simulink model "CMU_BORG_AplysiaModularNeuromechanics"  (R2024a)
settings: Solver=ode23  StartTime=0.0  StopTime=tend  FixedStep=0.001  MaxStep=0.1  RelTol=0.00001  AbsTol=0.0001
values from neighbouring files (symbols this model uses):
  B20_0 = 0    [ParameterRecalculation.m]    (also in ReferenceGeometry_and_Initialization.m)
  B31B32_0 = 0    [GetSteadyState.m]    (also in ParameterRecalculation.m = 1; ReferenceGeometry_and_Initialization.m = 1; VaryingSeaweedStrength.m = 1)
  B38_0 = 0    [ParameterRecalculation.m]    (also in ReferenceGeometry_and_Initialization.m)
  B40B30_0 = 0    [ParameterRecalculation.m]    (also in ReferenceGeometry_and_Initialization.m)
  B40B30_offTime_0 = 0    [ParameterRecalculation.m]    (also in ReferenceGeometry_and_Initialization.m)
  B43B45_0 = 0    [ParameterRecalculation.m]    (also in ReferenceGeometry_and_Initialization.m)
  B4B5_0 = 0    [ParameterRecalculation.m]    (also in ReferenceGeometry_and_Initialization.m)
  B64_0 = 1    [GetSteadyState.m]    (also in ParameterRecalculation.m = 0; ReferenceGeometry_and_Initialization.m = 0; VaryingSeaweedStrength.m = 0)
  B6B9B3_0 = 1    [GetSteadyState.m]    (also in ParameterRecalculation.m = 0; ReferenceGeometry_and_Initialization.m = 0; VaryingSeaweedStrength.m = 0)
  B7_0 = 0    [ParameterRecalculation.m]    (also in ReferenceGeometry_and_Initialization.m)
  B8_0 = 0    [ParameterRecalculation.m]    (also in ReferenceGeometry_and_Initialization.m)
  C1_0 = 0    [ParameterRecalculation.m]    (also in ReferenceGeometry_and_Initialization.m)
  C2_0 = 0    [ParameterRecalculation.m]    (also in ReferenceGeometry_and_Initialization.m)
  C6_0 = 0    [ParameterRecalculation.m]    (also in ReferenceGeometry_and_Initialization.m)
  C_theta = C_xg/(2*pi)    [ParameterRecalculation.m]    (also in ReferenceGeometry_and_Initialization.m = 0.000813600069086)
  C_xd = C_xg    [ParameterRecalculation.m]    (also in ReferenceGeometry_and_Initialization.m = 0.005112)
  C_xg = (1/inv_C(kk))*time_scaler*force_scaler    [DampingParameterConvergence.m]    (also in ReferenceGeometry_and_Initialization.m = 0.005112)
  C_xv = C_xd    [ParameterRecalculation.m]    (also in ReferenceGeometry_and_Initialization.m = 0.005112)
  C_yg = C_xg    [ParameterRecalculation.m]    (also in ReferenceGeometry_and_Initialization.m = 0.005112)
  CBI2_0 = 0    [ParameterRecalculation.m]    (also in ReferenceGeometry_and_Initialization.m)
  CBI3_0 = 0    [GetSteadyState.m]    (also in ParameterRecalculation.m = 1; ReferenceGeometry_and_Initialization.m = 1; VaryingSeaweedStrength.m = 1)
  CBI3_refractory_0 = 0    [ParameterRecalculation.m]    (also in ReferenceGeometry_and_Initialization.m)
  CBI3_stimOFF_0 = 0    [ParameterRecalculation.m]    (also in ReferenceGeometry_and_Initialization.m)
  CBI3_stimON_0 = 0    [ParameterRecalculation.m]    (also in ReferenceGeometry_and_Initialization.m)
  CBI4_0 = 0    [ParameterRecalculation.m]    (also in ReferenceGeometry_and_Initialization.m)
  E1_params = [AE10,TE10,tau_E1,L0_E1,Lmax_E1]    [ParameterRecalculation.m]    (also in ReferenceGeometry_and_Initialization.m)
  E2_params = [AE20,TE20,tau_E2,L0_E2,Lmax_E2]    [ParameterRecalculation.m]    (also in ReferenceGeometry_and_Initialization.m)
  E6_params = [AE60,TE60,tau_E6,L0_E6,Lmax_E6]    [ParameterRecalculation.m]    (also in ReferenceGeometry_and_Initialization.m)
  FE1_max = force_scaler*0.2    [ParameterRecalculation.m]    (also in ReferenceGeometry_and_Initialization.m = 0.048)
  FE2_max = FE1_max    [ParameterRecalculation.m]    (also in ReferenceGeometry_and_Initialization.m = 0.048)
  FE6_max = FE1_max    [ParameterRecalculation.m]    (also in ReferenceGeometry_and_Initialization.m = 0.048)
  FHinge_max = force_scaler*0.292    [ParameterRecalculation.m]    (also in ReferenceGeometry_and_Initialization.m = 0.07008)
  FI1d_max = force_scaler*3.2    [ParameterRecalculation.m]    (also in ReferenceGeometry_and_Initialization.m = 0.768)
  FI1v_max = FI1d_max    [ParameterRecalculation.m]    (also in ReferenceGeometry_and_Initialization.m = 0.768)
  FI2_max = force_scaler*1    [ParameterRecalculation.m]    (also in ReferenceGeometry_and_Initialization.m = 0.24)
  FI3_ant_max = force_scaler*0.1    [ParameterRecalculation.m]    (also in ReferenceGeometry_and_Initialization.m = 0.024)
  FI3_max = force_scaler*3    [ParameterRecalculation.m]    (also in ReferenceGeometry_and_Initialization.m = 0.72)
  FI4_max = force_scaler*0.9    [ParameterRecalculation.m]    (also in ReferenceGeometry_and_Initialization.m = 0.216)
  fixation_type = 0    [GetSteadyState.m]    (also in ModelController.m; VaryingSeaweedStrength.m)
  grasperR = 1    [ReferenceGeometry_and_Initialization.m]
  H_lumen = mean([L_jaw,L_LG]) / R_ref    [ReferenceGeometry_and_Initialization.m]
  Hinge_params = [A_hinge0,T_hinge0,tau_hinge,L0_hinge,Lmax_hinge]    [ParameterRecalculation.m]    (also in ReferenceGeometry_and_Initialization.m)
  I1d_params = [AI1d0,TI1d0,tau_I1d,L0_I1d,Lmax_I1d]    [ParameterRecalculation.m]    (also in ReferenceGeometry_and_Initialization.m)
  I1v_params = [AI1v0,TI1v0,tau_I1v,L0_I1v,Lmax_I1v]    [ParameterRecalculation.m]    (also in ReferenceGeometry_and_Initialization.m)
  I2_params = [AI20,TI20,tau_I2_ingestive,tau_I2_egestive,L0_I2,Lmax_I2]    [ParameterRecalculation.m]    (also in ReferenceGeometry_and_Initialization.m)
  I3_params = [AI30,TI30,tau_I3]    [ParameterRecalculation.m]    (also in ReferenceGeometry_and_Initialization.m)
  I3ant_params = [AI3_ant0,TI3_ant0,tau_I3ant]    [ParameterRecalculation.m]    (also in ReferenceGeometry_and_Initialization.m)
  I4_params = [AI40,TI40,tau_I4]    [ParameterRecalculation.m]    (also in ReferenceGeometry_and_Initialization.m)
  K_const = force_scaler*0.5    [ParameterRecalculation.m]    (also in ReferenceGeometry_and_Initialization.m = 0.12)
  K_Eso = force_scaler*0.01    [ParameterRecalculation.m]    (also in ReferenceGeometry_and_Initialization.m = 0.0024)
  K_H = force_scaler*2    [ParameterRecalculation.m]    (also in ReferenceGeometry_and_Initialization.m = 0.48)
  L0_eso = abs(xd0)    [ReferenceGeometry_and_Initialization.m]
  L0_H = 0    [ReferenceGeometry_and_Initialization.m]
  L0_I1d = L1d0    [ParameterRecalculation.m]    (also in ReferenceGeometry_and_Initialization.m)
  L0_I1v = L1v0    [ParameterRecalculation.m]    (also in ReferenceGeometry_and_Initialization.m)
  L_head = 0.82*tracing_scale_factor    [ReferenceGeometry_and_Initialization.m]
  MCC_0 = 1    [DampingParameterConvergence.m]    (also in ModelController.m; ParameterRecalculation.m = 0; ReferenceGeometry_and_Initialization.m = 0)
  params = param_vec    [ParameterRecalculation.m]    (also in ReferenceGeometry_and_Initialization.m)
  seaweed_strength = 1e6    (= 1000000)    [ModelController.m]    (also in VaryingSeaweedStrength.m = seaweed_strength_vec(ind))
  sens_chemical_lips = 0    [GetSteadyState.m]    (also in ModelController.m = 1; VaryingSeaweedStrength.m = 1)
  sens_mechanical_grasper = 1    [GetSteadyState.m]    (also in ModelController.m = 0; VaryingSeaweedStrength.m)
  sens_mechanical_lips = 1    [GetSteadyState.m]    (also in ModelController.m; VaryingSeaweedStrength.m)
  t_switch_chem_lips = 1e6    (= 1000000)    [GetSteadyState.m]    (also in ModelController.m = 54; VaryingSeaweedStrength.m)
  t_switch_fixation = 1e6    (= 1000000)    [GetSteadyState.m]    (also in ModelController.m = 30; VaryingSeaweedStrength.m = 4)
  t_switch_mech_grasp = 1e6    (= 1000000)    [GetSteadyState.m]    (also in ModelController.m = 10; VaryingSeaweedStrength.m)
  t_switch_mech_lips = 1e6    (= 1000000)    [GetSteadyState.m]    (also in ModelController.m; VaryingSeaweedStrength.m)
  theta_fg = buccal_mass_data(7)    [PlotModel.m]    (also in ReferenceGeometry_and_Initialization.m = -(head_outline{4,"Angle"} - head_outline{3,"Angle"})*(pi/180)
  theta_g0 = (180-(head_outline{3,"Angle"} + rot_global +5))*(pi/180)    [ReferenceGeometry_and_Initialization.m]
  theta_H = buccal_mass_data(6)    [PlotModel.m]    (also in ReferenceGeometry_and_Initialization.m = pi + theta_H_tilde - theta_g0)
  time_scaler = 1    [DampingParameterConvergence.m]    (also in ReferenceGeometry_and_Initialization.m = 1.065)
  ukg = 0.95*usg    (= 0.95)    [ParameterRecalculation.m]    (also in ReferenceGeometry_and_Initialization.m)
  ukh = 0.75*ush    (= 0.75)    [ParameterRecalculation.m]    (also in ReferenceGeometry_and_Initialization.m)
  usg = 1    [ParameterRecalculation.m]    (also in ReferenceGeometry_and_Initialization.m)
  ush = 1    [ParameterRecalculation.m]    (also in ReferenceGeometry_and_Initialization.m)
  xd0 = L_head - L1d0    [ReferenceGeometry_and_Initialization.m]
  xg0 = L_head + L_CG * cosd(a_CG) + 0.3    [ReferenceGeometry_and_Initialization.m]
  xh0 = 0    [ReferenceGeometry_and_Initialization.m]
  xv0 = L_head - L1v0    [ReferenceGeometry_and_Initialization.m]
  yg0 = L_CG * sind(a_CG) + 0.4    [ReferenceGeometry_and_Initialization.m]
(part 1 of 4)
settings Model: SimulationMode=accelerator  Creator=MichaelBennington  LastModifiedBy=MichaelBennington
settings SolverCC: ZeroCrossControl=DisableAll  ZeroCrossAlgorithm=Adaptive
settings OptimizationCC: ReuseModelBlockBuffer=off
settings DebuggingCC: IgnoredZcDiagnostic=none
settings RTWCC: GPUComputeCapability=3.5

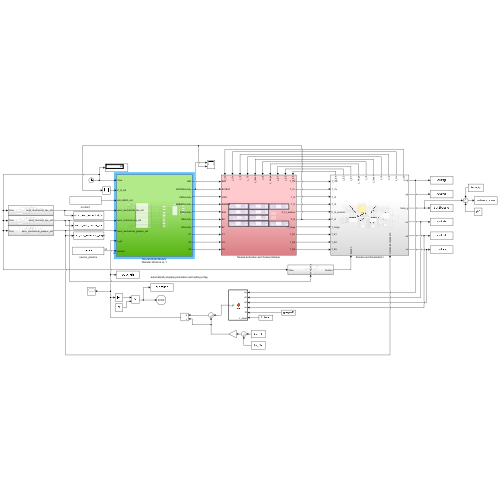
[thumbnail: Simulink's stored preview of the top-level diagram]
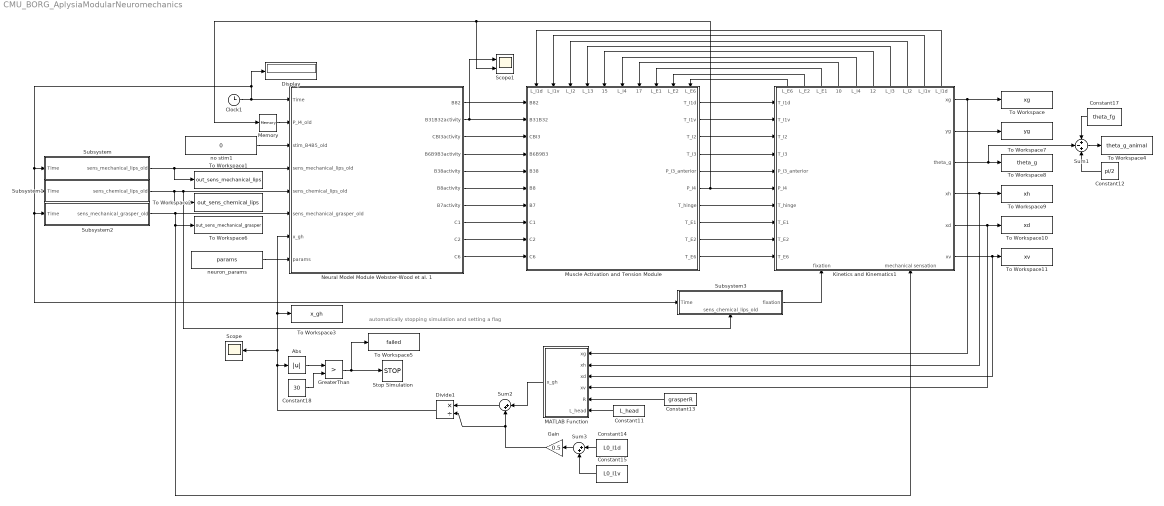
== system CMU_BORG_AplysiaModularNeuromechanics ==
  note: automatically stopping simulation and setting a flag
  Abs : Abs  SaturateOnIntegerOverflow=off
  Clock1 : Clock
  Constant11 : Constant  Value=L_head
  Constant12 : Constant  Value=pi/2
  Constant13 : Constant  Value=grasperR
  Constant14 : Constant  Value=L0_I1d
  Constant15 : Constant  Value=L0_I1v
  Constant17 : Constant  Value=theta_fg
  Constant18 : Constant  Value=30
  Display : Display
  Divide1 : Product  Inputs=*/
  Gain : Gain  Gain=0.5
  GreaterThan : RelationalOperator  Operator=>  OutDataTypeStr=boolean  RndMeth=Simplest  InputSameDT=off
  Kinetics and Kinematics1 : Subsystem
      settings: PortSchema="{\"entries\":[{\"content\":{\"sides\":[{\"content\":{\"connectorIds\":[\"In1\",\"In2\",\"In3\",\"In4\",\"In5\",\"In6\",\"In7\",\"In8\",\"In9\",\"In10\"]},\"type\":\"ConnectorPlacement.EquallySpacedRectSide\",\"uuid\":\"feb973b9-0be4-4875-8bab-e7ecafe4ce91\"},{\"content\":{\"connectorIds\":[\"Out1\",\"Out2\",\"Out3\",\"Out4\",\"Out5\",\"Out6\"],\"side\":\"RIGHT\"},\"type\":\"ConnectorPlacement.EquallySpacedRectSide\",\"uuid\":\"c5092c36-404e-4254-bef3-0d67bb5be9d9\"},{\"content\":{\"connectorIds\":[\"Out7\",\"Out8\",\"Out9\",\"Out10\",\"Out11\",\"Out12\",\"Out13\",\"Out14\",\"Out15\",\"Out16\"],\"side\":\"TOP\"},\"type\":\"ConnectorPlacement.EquallySpacedRectSide\",\"uuid\":\"bd9119a0-4095-4707-a24a-63f80d66a5e2\"},{\"content\":{\"connectorIds\":[\"In11\",\"In12\"],\"side\":\"BOTTOM\"},\"type\":\"ConnectorPlacement.EquallySpacedRectSide\",\"uuid\":\"ad89abb6-7f53-48b7-b4f1-a6034e6f6b49\"}]},\"type\":\"ConnectorPlacement.EquallySpacedConnector\",\"uuid\":\"6bece42c-f05e-4dc2-8f2f-f52897a5dfb1\"}],\"packageUris\":[\"http://schema.mathworks.com/mf0/Connector/R2020b\"],\"version\":\"1.0\"}"
  MATLAB Function : MATLAB Function  TreatAsAtomicUnit=on
  Memory : Memory
  Muscle Activation and Tension Module : Subsystem
      settings: PortSchema="{\"entries\":[{\"content\":{\"sides\":[{\"content\":{\"connectorIds\":[\"In1\",\"In2\",\"In3\",\"In4\",\"In5\",\"In6\",\"In7\",\"In8\",\"In9\",\"In10\"]},\"type\":\"ConnectorPlacement.EquallySpacedRectSide\",\"uuid\":\"3ed42070-edfc-4f7d-bbc9-5418b4631d85\"},{\"content\":{\"connectorIds\":[\"Out1\",\"Out2\",\"Out3\",\"Out4\",\"Out5\",\"Out6\",\"Out7\",\"Out8\",\"Out9\",\"Out10\"],\"side\":\"RIGHT\"},\"type\":\"ConnectorPlacement.EquallySpacedRectSide\",\"uuid\":\"9529d621-06eb-4de0-be68-068c8ead65ac\"},{\"content\":{\"connectorIds\":[\"In11\",\"In12\",\"In13\",\"In14\",\"In15\",\"In16\",\"In17\",\"In18\",\"In19\",\"In20\"],\"side\":\"TOP\"},\"type\":\"ConnectorPlacement.EquallySpacedRectSide\",\"uuid\":\"028e6ff9-8ac1-449c-b22e-a0a954505d61\"}]},\"type\":\"ConnectorPlacement.EquallySpacedConnector\",\"uuid\":\"edcba6fa-e4ae-48e3-a50b-df7cd108ff35\"}],\"packageUris\":[\"http://schema.mathworks.com/mf0/Connector/R2020b\"],\"version\":\"1.0\"}"
  Neural Model Module Webster-Wood et al. 1 : Subsystem
  Scope : Scope
  Scope1 : Scope  NumInputPorts=2
  Stop Simulation : Stop
  Subsystem : Subsystem
  Subsystem1 : Subsystem
  Subsystem2 : Subsystem
  Subsystem3 : Subsystem
      settings: PortSchema="{\"entries\":[{\"content\":{\"sides\":[{\"content\":{\"connectorIds\":[\"In1\"]},\"type\":\"ConnectorPlacement.EquallySpacedRectSide\",\"uuid\":\"4db34430-399f-4704-aacb-c58121948b76\"},{\"content\":{\"connectorIds\":[\"Out1\"],\"side\":\"RIGHT\"},\"type\":\"ConnectorPlacement.EquallySpacedRectSide\",\"uuid\":\"b1912424-5bc4-479d-9601-ca1764a05c0d\"},{\"content\":{\"connectorIds\":[],\"side\":\"TOP\"},\"type\":\"ConnectorPlacement.EquallySpacedRectSide\",\"uuid\":\"e34c704c-48ea-4069-bc3f-08ffaf2b3e65\"},{\"content\":{\"connectorIds\":[\"In2\"],\"side\":\"BOTTOM\"},\"type\":\"ConnectorPlacement.EquallySpacedRectSide\",\"uuid\":\"845d24db-429a-4efd-80d9-e92f93226b00\"}]},\"type\":\"ConnectorPlacement.EquallySpacedConnector\",\"uuid\":\"7cfd80de-20d7-4cb7-a610-d527eb736c28\"}],\"packageUris\":[\"http://schema.mathworks.com/mf0/Connector/R2020b\"],\"version\":\"1.0\"}"
  Sum1 : Sum  Inputs=+-+
  Sum2 : Sum  Inputs=|++
  Sum3 : Sum  Inputs=|++
  To Workspace : ToWorkspace  VariableName=xg  SampleTime=-1
  To Workspace1 : ToWorkspace  VariableName=out_sens_mechanical_lips  SampleTime=-1
  To Workspace10 : ToWorkspace  VariableName=xd  SampleTime=-1
  To Workspace11 : ToWorkspace  VariableName=xv  SampleTime=-1
  To Workspace2 : ToWorkspace  VariableName=out_sens_chemical_lips  SampleTime=-1
  To Workspace3 : ToWorkspace  VariableName=x_gh  SampleTime=-1
  To Workspace4 : ToWorkspace  VariableName=theta_g_animal  SampleTime=-1
  To Workspace5 : ToWorkspace  VariableName=failed  SampleTime=-1
  To Workspace6 : ToWorkspace  VariableName=out_sens_mechanical_grasper  SampleTime=-1
  To Workspace7 : ToWorkspace  VariableName=yg  SampleTime=-1
  To Workspace8 : ToWorkspace  VariableName=theta_g  SampleTime=-1
  To Workspace9 : ToWorkspace  VariableName=xh  SampleTime=-1
  neuron_params : Constant  Value=params
  no stim1 : Constant  Value=0
  wires:
  no stim1/1 -> Neural Model Module Webster-Wood et al. 1/3(stim_B4B5_old)
  Subsystem2/1(sens_mechanical_grasper_old) -> To Workspace6/1, Kinetics and Kinematics1/12(mechanical sensation), Neural Model Module Webster-Wood et al. 1/6(sens_mechanical_grasper_old)
  Subsystem3/1(fixation) -> Kinetics and Kinematics1/11(fixation)
  Kinetics and Kinematics1/7(L_E6) -> Muscle Activation and Tension Module/20(L_E6)
  Kinetics and Kinematics1/8(L_E2) -> Muscle Activation and Tension Module/19(L_E2)
  Kinetics and Kinematics1/9(L_E1) -> Muscle Activation and Tension Module/18(L_E1)
  Kinetics and Kinematics1/10(L_hinge) -> Muscle Activation and Tension Module/17(L_hinge)
  Kinetics and Kinematics1/11(L_I4) -> Muscle Activation and Tension Module/16(L_I4)
  Kinetics and Kinematics1/12(L_I3ant) -> Muscle Activation and Tension Module/15(L_I3ant)
  Kinetics and Kinematics1/13(L_I3) -> Muscle Activation and Tension Module/14(L_13)
  Kinetics and Kinematics1/14(L_I2) -> Muscle Activation and Tension Module/13(L_I2)
  Kinetics and Kinematics1/15(L_I1v) -> Muscle Activation and Tension Module/12(L_I1v)
  Kinetics and Kinematics1/16(L_I1d) -> Muscle Activation and Tension Module/11(L_I1d)
  Clock1/1 -> Subsystem1/1(Time), Subsystem3/1(Time), Subsystem2/1(Time), Subsystem/1(Time), Display/1, Neural Model Module Webster-Wood et al. 1/1(Time)
  Memory/1 -> Neural Model Module Webster-Wood et al. 1/2(P_I4_old)
  Kinetics and Kinematics1/1(xg) -> To Workspace/1, MATLAB Function/1(xg)
  Kinetics and Kinematics1/2(yg) -> To Workspace7/1
  Kinetics and Kinematics1/3(theta_g) -> Sum1/2, To Workspace8/1
  Kinetics and Kinematics1/4(xh) -> MATLAB Function/2(xh), To Workspace9/1
  Kinetics and Kinematics1/5(xd) -> MATLAB Function/4(xv), To Workspace10/1
  Kinetics and Kinematics1/6(xv) -> MATLAB Function/3(xd), To Workspace11/1
  Muscle Activation and Tension Module/1(T_I1d) -> Kinetics and Kinematics1/1(T_I1d)
  Muscle Activation and Tension Module/2(T_I1v) -> Kinetics and Kinematics1/2(T_I1v)
  Muscle Activation and Tension Module/3(T_I2) -> Kinetics and Kinematics1/3(T_I2)
  Muscle Activation and Tension Module/4(T_I3) -> Kinetics and Kinematics1/4(T_I3)
  Muscle Activation and Tension Module/5(P_I3_anterior) -> Kinetics and Kinematics1/5(P_I3_anterior)
  Muscle Activation and Tension Module/6(P_I4) -> Kinetics and Kinematics1/6(P_I4), Scope1/2, Memory/1
  Muscle Activation and Tension Module/7(T_hinge) -> Kinetics and Kinematics1/7(T_hinge)
  Muscle Activation and Tension Module/8(T_E1) -> Kinetics and Kinematics1/8(T_E1)
  Muscle Activation and Tension Module/9(T_E2) -> Kinetics and Kinematics1/9(T_E2)
  Muscle Activation and Tension Module/10(T_E6) -> Kinetics and Kinematics1/10(T_E6)
  Neural Model Module Webster-Wood et al. 1/2(B31B32activity) -> Scope1/1, Muscle Activation and Tension Module/2(B31B32)
  Neural Model Module Webster-Wood et al. 1/3(CBI3activity) -> Muscle Activation and Tension Module/3(CBI3)
  Neural Model Module Webster-Wood et al. 1/4(B6B9B3activity) -> Muscle Activation and Tension Module/4(B6B9B3)
  Neural Model Module Webster-Wood et al. 1/5(B38activity) -> Muscle Activation and Tension Module/5(B38)
  Neural Model Module Webster-Wood et al. 1/6(B8activity) -> Muscle Activation and Tension Module/6(B8)
  Neural Model Module Webster-Wood et al. 1/7(B7activity) -> Muscle Activation and Tension Module/7(B7)
  Neural Model Module Webster-Wood et al. 1/1(B82) -> Muscle Activation and Tension Module/1(B82)
  Neural Model Module Webster-Wood et al. 1/10(C6) -> Muscle Activation and Tension Module/10(C6)
  Neural Model Module Webster-Wood et al. 1/9(C2) -> Muscle Activation and Tension Module/9(C2)
  Neural Model Module Webster-Wood et al. 1/8(C1) -> Muscle Activation and Tension Module/8(C1)
  Constant11/1 -> MATLAB Function/6(L_head)
  Constant13/1 -> MATLAB Function/5(R)
  Constant14/1 -> Sum3/1
  Constant15/1 -> Sum3/2
  Sum3/1 -> Gain/1
  Sum2/1 -> Divide1/1
  Divide1/1 -> Neural Model Module Webster-Wood et al. 1/7(x_gh), To Workspace3/1, Scope/1, Abs/1
  Gain/1 -> Sum2/2, Divide1/2
  MATLAB Function/1(x_gh) -> Sum2/1
  Constant12/1 -> Sum1/3
  GreaterThan/1 -> Stop Simulation/1, To Workspace5/1
  Constant18/1 -> GreaterThan/2
  Abs/1 -> GreaterThan/1
  neuron_params/1 -> Neural Model Module Webster-Wood et al. 1/8(params)
  Sum1/1 -> To Workspace4/1
  Constant17/1 -> Sum1/1
  Subsystem/1(sens_mechanical_lips_old) -> To Workspace1/1, Neural Model Module Webster-Wood et al. 1/4(sens_mechanical_lips_old)
  Subsystem1/1(sens_chemical_lips_old) -> Subsystem3/2(sens_chemical_lips_old), Neural Model Module Webster-Wood et al. 1/5(sens_chemical_lips_old), To Workspace2/1

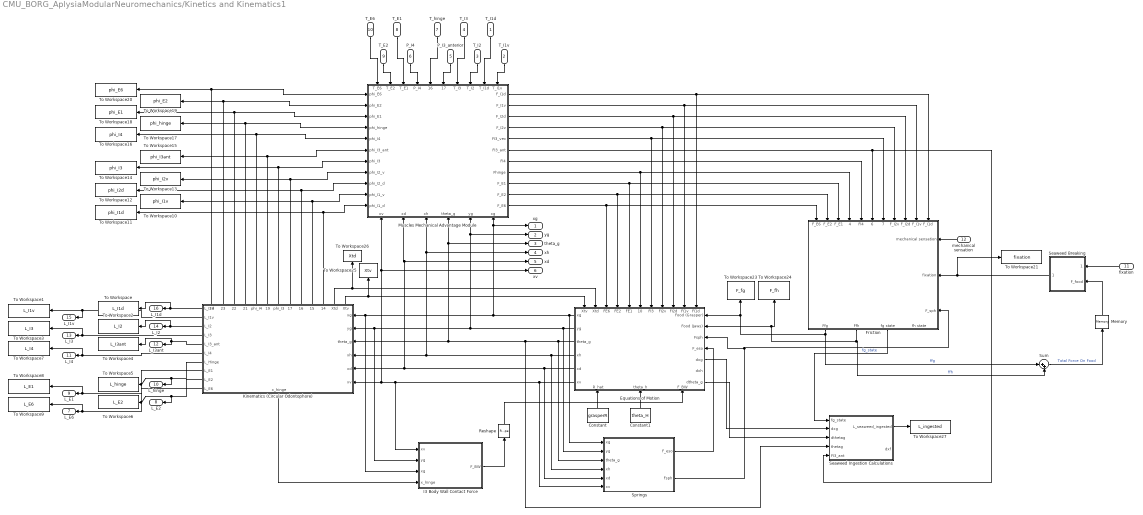
== system CMU_BORG_AplysiaModularNeuromechanics/Kinetics and Kinematics1 ==
  T_I1d : Inport
  T_I1v : Inport  Port=2
  T_I2 : Inport  Port=3
  T_I3 : Inport  Port=4
  P_I3_anterior : Inport  Port=5
  P_I4 : Inport  Port=6
  T_hinge : Inport  Port=7
  T_E1 : Inport  Port=8
  T_E2 : Inport  Port=9
  T_E6 : Inport  Port=10
  fixation : Inport  Port=11
  mechanical sensation : Inport  Port=12
  Constant : Constant  Value=grasperR
  Constant1 : Constant  Value=theta_H
  Equations of Motion : Subsystem
      settings: PortSchema="{\"entries\":[{\"content\":{\"sides\":[{\"content\":{\"connectorIds\":[\"In1\",\"In2\",\"In3\",\"In4\",\"Out7\",\"Out8\",\"Out9\"]},\"type\":\"ConnectorPlacement.EquallySpacedRectSide\",\"uuid\":\"fc8d0afd-02a2-478d-bf19-33a99a16df05\"},{\"content\":{\"connectorIds\":[\"Out1\",\"Out2\",\"Out3\",\"Out4\",\"Out5\",\"Out6\"],\"side\":\"RIGHT\"},\"type\":\"ConnectorPlacement.EquallySpacedRectSide\",\"uuid\":\"2253c95e-6db7-473c-a5d6-d56fdecd2583\"},{\"content\":{\"connectorIds\":[\"In5\",\"In6\",\"In7\",\"In8\",\"In9\",\"In10\",\"In11\",\"In12\",\"In13\",\"In14\",\"In15\"],\"side\":\"TOP\"},\"type\":\"ConnectorPlacement.EquallySpacedRectSide\",\"uuid\":\"0ccf99ea-7251-4d75-8ccd-da18da8d2aef\"},{\"content\":{\"connectorIds\":[\"In16\",\"In17\",\"In18\"],\"side\":\"BOTTOM\"},\"type\":\"ConnectorPlacement.EquallySpacedRectSide\",\"uuid\":\"d224286b-c4b9-4c0b-afff-0678c6181b4d\"}]},\"type\":\"ConnectorPlacement.EquallySpacedConnector\",\"uuid\":\"96948490-78d0-4299-9707-28e1bc260310\"}],\"packageUris\":[\"http://schema.mathworks.com/mf0/Connector/R2020b\"],\"version\":\"1.0\"}"
  Friction : Subsystem
      settings: PortSchema="{\"entries\":[{\"content\":{\"sides\":[{\"content\":{\"connectorIds\":[\"In1\",\"In2\",\"In3\",\"In4\",\"In5\",\"In6\",\"In7\",\"In8\",\"In9\",\"In10\",\"In11\"]},\"type\":\"ConnectorPlacement.EquallySpacedRectSide\",\"uuid\":\"97b41599-dff3-491f-acd3-dab3384a422d\"},{\"content\":{\"connectorIds\":[\"Out1\",\"Out2\",\"Out3\",\"Out4\"],\"side\":\"RIGHT\"},\"type\":\"ConnectorPlacement.EquallySpacedRectSide\",\"uuid\":\"7a9b386b-0421-4afc-b8c2-6f24613cda45\"},{\"content\":{\"connectorIds\":[],\"side\":\"TOP\"},\"type\":\"ConnectorPlacement.EquallySpacedRectSide\",\"uuid\":\"b6a8e481-ded8-4250-a21f-c0166a430c6b\"},{\"content\":{\"connectorIds\":[\"In12\",\"In13\",\"In14\"],\"side\":\"BOTTOM\"},\"type\":\"ConnectorPlacement.EquallySpacedRectSide\",\"uuid\":\"d5796b21-30a2-4a10-961b-04e48d1aad8b\"}]},\"type\":\"ConnectorPlacement.EquallySpacedConnector\",\"uuid\":\"b13cf459-4587-426d-a5d2-bd8c478a3c8b\"}],\"packageUris\":[\"http://schema.mathworks.com/mf0/Connector/R2020b\"],\"version\":\"1.0\"}"
  I3 Body Wall Contact Force : Subsystem
  Kinematics (Circular Odontophore) : Subsystem
      settings: PortSchema="{\"entries\":[{\"content\":{\"sides\":[{\"content\":{\"connectorIds\":[\"In1\",\"In2\",\"In3\",\"In4\",\"In5\",\"In6\"]},\"type\":\"ConnectorPlacement.EquallySpacedRectSide\",\"uuid\":\"9a4ef7c8-abc6-448b-bb3a-4c454413f116\"},{\"content\":{\"connectorIds\":[\"Out1\",\"Out2\",\"Out3\",\"Out4\",\"Out5\",\"Out6\",\"Out7\",\"Out8\",\"Out9\",\"Out10\"],\"side\":\"RIGHT\"},\"type\":\"ConnectorPlacement.EquallySpacedRectSide\",\"uuid\":\"3afa5e1b-061c-428a-a585-6f6007c5b0dc\"},{\"content\":{\"connectorIds\":[\"Out12\",\"Out13\",\"Out14\",\"Out15\",\"Out16\",\"Out17\",\"Out18\",\"Out19\",\"Out20\",\"Out21\",\"Out22\",\"Out23\",\"Out24\"],\"side\":\"TOP\"},\"type\":\"ConnectorPlacement.EquallySpacedRectSide\",\"uuid\":\"ec112a13-881a-4563-8a11-697c316b2d4f\"},{\"content\":{\"connectorIds\":[\"Out11\"],\"side\":\"BOTTOM\"},\"type\":\"ConnectorPlacement.EquallySpacedRectSide\",\"uuid\":\"763b50d4-e3e7-45b9-9ae3-aa70a1782eba\"}]},\"type\":\"ConnectorPlacement.EquallySpacedConnector\",\"uuid\":\"2b7d157a-c6a5-494b-9033-60740e92ca72\"}],\"packageUris\":[\"http://schema.mathworks.com/mf0/Connector/R2020b\"],\"version\":\"1.0\"}"
  Memory : Memory
  Muscles Mechanical Advantage Module : Subsystem
      settings: PortSchema="{\"entries\":[{\"content\":{\"sides\":[{\"content\":{\"connectorIds\":[\"In1\",\"In2\",\"In3\",\"In4\",\"In5\",\"In6\",\"In7\",\"In8\",\"In9\",\"In10\",\"In11\"]},\"type\":\"ConnectorPlacement.EquallySpacedRectSide\",\"uuid\":\"a912b0e9-42ce-449b-a797-141e8809ae90\"},{\"content\":{\"connectorIds\":[\"Out1\",\"Out2\",\"Out3\",\"Out4\",\"Out5\",\"Out6\",\"Out7\",\"Out8\",\"Out9\",\"Out10\",\"Out11\"],\"side\":\"RIGHT\"},\"type\":\"ConnectorPlacement.EquallySpacedRectSide\",\"uuid\":\"77531ae2-3784-4c4f-a31c-3289419d6da8\"},{\"content\":{\"connectorIds\":[\"In12\",\"In13\",\"In14\",\"In15\",\"In16\",\"In17\",\"In18\",\"In19\",\"In20\",\"In21\"],\"side\":\"TOP\"},\"type\":\"ConnectorPlacement.EquallySpacedRectSide\",\"uuid\":\"297c6c95-5c55-462e-90e8-7195e38b8668\"},{\"content\":{\"connectorIds\":[\"In22\",\"In23\",\"In24\",\"In25\",\"In26\",\"In27\"],\"side\":\"BOTTOM\"},\"type\":\"ConnectorPlacement.EquallySpacedRectSide\",\"uuid\":\"47d39c31-e857-46ee-b2b8-51c31c90f011\"}]},\"type\":\"ConnectorPlacement.EquallySpacedConnector\",\"uuid\":\"67a8826f-c33f-429f-90c6-68e25a4513f3\"}],\"packageUris\":[\"http://schema.mathworks.com/mf0/Connector/R2020b\"],\"version\":\"1.0\"}"
  Reshape : Reshape  OutputDimensionality=Customize  OutputDimensions=2
  Seaweed Breaking : Subsystem
  Seaweed Ingestion Calculations : Subsystem
  Springs : Subsystem
  Sum : Sum  Inputs=|++
  To Workspace : ToWorkspace  VariableName=L_I1d  SampleTime=-1
  To Workspace1 : ToWorkspace  VariableName=L_I1v  SampleTime=-1
  To Workspace10 : ToWorkspace  VariableName=phi_I1v  SampleTime=-1
  To Workspace11 : ToWorkspace  VariableName=phi_I1d  SampleTime=-1
  To Workspace12 : ToWorkspace  VariableName=phi_I2d  SampleTime=-1
  To Workspace13 : ToWorkspace  VariableName=phi_I2v  SampleTime=-1
  To Workspace14 : ToWorkspace  VariableName=phi_I3  SampleTime=-1
  To Workspace15 : ToWorkspace  VariableName=phi_I3ant  SampleTime=-1
  To Workspace16 : ToWorkspace  VariableName=phi_I4  SampleTime=-1
  To Workspace17 : ToWorkspace  VariableName=phi_hinge  SampleTime=-1
  To Workspace18 : ToWorkspace  VariableName=phi_E1  SampleTime=-1
  To Workspace19 : ToWorkspace  VariableName=phi_E2  SampleTime=-1
  To Workspace2 : ToWorkspace  VariableName=L_I2  SampleTime=-1
  To Workspace20 : ToWorkspace  VariableName=phi_E6  SampleTime=-1
  To Workspace21 : ToWorkspace  VariableName=fixation  SampleTime=-1
  To Workspace23 : ToWorkspace  VariableName=F_fg  SampleTime=-1
  To Workspace24 : ToWorkspace  VariableName=F_fh  SampleTime=-1
  To Workspace25 : ToWorkspace  VariableName=Xtv  SampleTime=-1
  To Workspace26 : ToWorkspace  VariableName=Xtd  SampleTime=-1
  To Workspace27 : ToWorkspace  VariableName=L_ingested  SampleTime=-1
  To Workspace3 : ToWorkspace  VariableName=L_I3  SampleTime=-1
  To Workspace4 : ToWorkspace  VariableName=L_I3ant  SampleTime=-1
  To Workspace5 : ToWorkspace  VariableName=L_hinge  SampleTime=-1
  To Workspace6 : ToWorkspace  VariableName=L_E2  SampleTime=-1
  To Workspace7 : ToWorkspace  VariableName=L_I4  SampleTime=-1
  To Workspace8 : ToWorkspace  VariableName=L_E1  SampleTime=-1
  To Workspace9 : ToWorkspace  VariableName=L_E6  SampleTime=-1
  xg : Outport
  yg : Outport  Port=2
  theta_g : Outport  Port=3
  xh : Outport  Port=4
  xd : Outport  Port=5
  xv : Outport  Port=6
  L_E6 : Outport  Port=7
  L_E2 : Outport  Port=8
  L_E1 : Outport  Port=9
  L_hinge : Outport  Port=10
  L_I4 : Outport  Port=11
  L_I3ant : Outport  Port=12
  L_I3 : Outport  Port=13
  L_I2 : Outport  Port=14
  L_I1v : Outport  Port=15
  L_I1d : Outport  Port=16
  wires:
  Friction/1(Ffg) -> Equations of Motion/1(Food (Grasper)), To Workspace23/1, Sum/1  "ffg"
  Equations of Motion/1(xg) -> Springs/1(xg), I3 Body Wall Contact Force/3(xg), Kinematics (Circular Odontophore)/1(xg), xg/1, Muscles Mechanical Advantage Module/27(xg)
  Equations of Motion/2(yg) -> Springs/2(yg), I3 Body Wall Contact Force/2(yg), Kinematics (Circular Odontophore)/2(yg), yg/1, Muscles Mechanical Advantage Module/26(yg)
  Equations of Motion/3(theta_g) -> Springs/3(theta_g), Seaweed Ingestion Calculations/4(thetag), Kinematics (Circular Odontophore)/3(theta_g), theta_g/1, Muscles Mechanical Advantage Module/25(theta_g)
  Equations of Motion/4(xh) -> Springs/4(xh), Kinematics (Circular Odontophore)/4(xh), xh/1, Muscles Mechanical Advantage Module/24(xh)
  Equations of Motion/5(xd) -> Springs/5(xd), Kinematics (Circular Odontophore)/5(xd), xd/1, Muscles Mechanical Advantage Module/23(xd)
  Equations of Motion/6(xv) -> Springs/6(xv), Kinematics (Circular Odontophore)/6(xv), xv/1, Muscles Mechanical Advantage Module/22(xv), I3 Body Wall Contact Force/1(xv)
  Kinematics (Circular Odontophore)/1(L_I1d) -> To Workspace/1, L_I1d/1
  Kinematics (Circular Odontophore)/2(L_I1v) -> L_I1v/1, To Workspace1/1
  Kinematics (Circular Odontophore)/3(L_I2) -> To Workspace2/1, L_I2/1
  Kinematics (Circular Odontophore)/4(L_I3) -> To Workspace3/1, L_I3/1
  Kinematics (Circular Odontophore)/6(L_I4) -> To Workspace7/1, L_I4/1
  Kinematics (Circular Odontophore)/5(L_I3_ant) -> L_I3ant/1, To Workspace4/1
  Kinematics (Circular Odontophore)/7(L_Hinge) -> L_hinge/1, To Workspace5/1
  Kinematics (Circular Odontophore)/8(L_E1) -> To Workspace8/1, L_E1/1
  Kinematics (Circular Odontophore)/9(L_E2) -> L_E2/1, To Workspace6/1
  Kinematics (Circular Odontophore)/10(L_E6) -> To Workspace9/1, L_E6/1
  Kinematics (Circular Odontophore)/24(phi_E6) -> Muscles Mechanical Advantage Module/1(phi_E6), To Workspace20/1
  Kinematics (Circular Odontophore)/23(phi_E2) -> Muscles Mechanical Advantage Module/2(phi_E2), To Workspace19/1
  Kinematics (Circular Odontophore)/22(phi_E1) -> Muscles Mechanical Advantage Module/3(phi_E1), To Workspace18/1
  Kinematics (Circular Odontophore)/20(phi_I4) -> Muscles Mechanical Advantage Module/5(phi_I4), To Workspace16/1
  Kinematics (Circular Odontophore)/19(phi_I3_ant) -> Muscles Mechanical Advantage Module/6(phi_I3_ant), To Workspace15/1
  Kinematics (Circular Odontophore)/18(phi_I3) -> Muscles Mechanical Advantage Module/7(phi_I3), To Workspace14/1
  Kinematics (Circular Odontophore)/17(phi_I2v) -> Muscles Mechanical Advantage Module/8(phi_I2_v), To Workspace13/1
  Kinematics (Circular Odontophore)/16(phi_I2d) -> Muscles Mechanical Advantage Module/9(phi_I2_d), To Workspace12/1
  Kinematics (Circular Odontophore)/15(phi_I1v) -> Muscles Mechanical Advantage Module/10(phi_I1_v), To Workspace10/1
  Kinematics (Circular Odontophore)/14(phi_I1d) -> Muscles Mechanical Advantage Module/11(phi_I1_d), To Workspace11/1
  Muscles Mechanical Advantage Module/10(F_E2) -> Equations of Motion/12(FE2), Friction/2(F_E2)
  Muscles Mechanical Advantage Module/9(F_E1) -> Equations of Motion/11(FE1), Friction/3(F_E1)
  Muscles Mechanical Advantage Module/8(Fhinge) -> Equations of Motion/10(Fhinge), Friction/4(Fhinge)
  Muscles Mechanical Advantage Module/5(FI3_vec) -> Friction/7(FI3_vec), Equations of Motion/9(FI3)
  Muscles Mechanical Advantage Module/4(F_I2v) -> Equations of Motion/8(FI2v), Friction/8(F_I2v)
  Muscles Mechanical Advantage Module/3(F_I2d) -> Friction/9(F_I2d), Equations of Motion/7(FI2d)
  Muscles Mechanical Advantage Module/2(F_I1v) -> Friction/10(F_I1v), Equations of Motion/6(FI1v)
  Muscles Mechanical Advantage Module/1(F_I1d) -> Friction/11(F_I1d), Equations of Motion/5(FI1d)
  Springs/2(Fsph) -> Equations of Motion/3(Fsph), Friction/14(F_sph)
  Springs/1(F_eso) -> Equations of Motion/4(F_eso)
  mechanical sensation/1 -> Friction/12(mechanical sensation)
  T_I2/1 -> Muscles Mechanical Advantage Module/19(T_I2)
  T_I3/1 -> Muscles Mechanical Advantage Module/18(T_I3)
  P_I3_anterior/1 -> Muscles Mechanical Advantage Module/17(P_I3_ant)
  T_hinge/1 -> Muscles Mechanical Advantage Module/16(T_hinge)
  P_I4/1 -> Muscles Mechanical Advantage Module/15(P_I4)
  T_E1/1 -> Muscles Mechanical Advantage Module/14(T_E1)
  T_E2/1 -> Muscles Mechanical Advantage Module/13(T_E2)
  T_E6/1 -> Muscles Mechanical Advantage Module/12(T_E6)
  Friction/2(Ffh) -> To Workspace24/1, Equations of Motion/2(Food (Jaws)), Sum/2  "ffh"
  Kinematics (Circular Odontophore)/12(Xtv) -> Equations of Motion/15(Xtv), To Workspace25/1
  Kinematics (Circular Odontophore)/13(Xtd) -> Equations of Motion/14(Xtd), To Workspace26/1
  Muscles Mechanical Advantage Module/7(FI4) -> Friction/5(FI4)
  Muscles Mechanical Advantage Module/6(FI3_ant) -> Seaweed Ingestion Calculations/5(FI3_ant), Friction/6(PI3_ant)
  Muscles Mechanical Advantage Module/11(F_E6) -> Equations of Motion/13(FE6), Friction/1(F_E6)
  Kinematics (Circular Odontophore)/21(phi_Hinge) -> Muscles Mechanical Advantage Module/4(phi_hinge), To Workspace17/1
  T_I1d/1 -> Muscles Mechanical Advantage Module/20(T_I1d)
  T_I1v/1 -> Muscles Mechanical Advantage Module/21(T_I1v)
  Equations of Motion/7(dxg) -> Seaweed Ingestion Calculations/2(dxg)
  Equations of Motion/9(dtheta_g) -> Seaweed Ingestion Calculations/3(dthetag)
  Friction/3(fg state) -> Seaweed Ingestion Calculations/1(fg_state)  "fg_state"
  Seaweed Ingestion Calculations/1(L_seaweed_ingested) -> To Workspace27/1
  Constant/1 -> Equations of Motion/18(R_hat)
  Constant1/1 -> Equations of Motion/17(theta_h)
  Kinematics (Circular Odontophore)/11(x_hinge) -> I3 Body Wall Contact Force/4(x_hinge)
  I3 Body Wall Contact Force/1(F_BW) -> Reshape/1
  Reshape/1 -> Equations of Motion/16(F_BW)
  Sum/1 -> Memory/1  "Total Force On Food"
  fixation/1 -> Seaweed Breaking/1(fixation)
  Seaweed Breaking/1(fixation_out) -> To Workspace21/1, Friction/13(fixation)
  Memory/1 -> Seaweed Breaking/2(F_food)

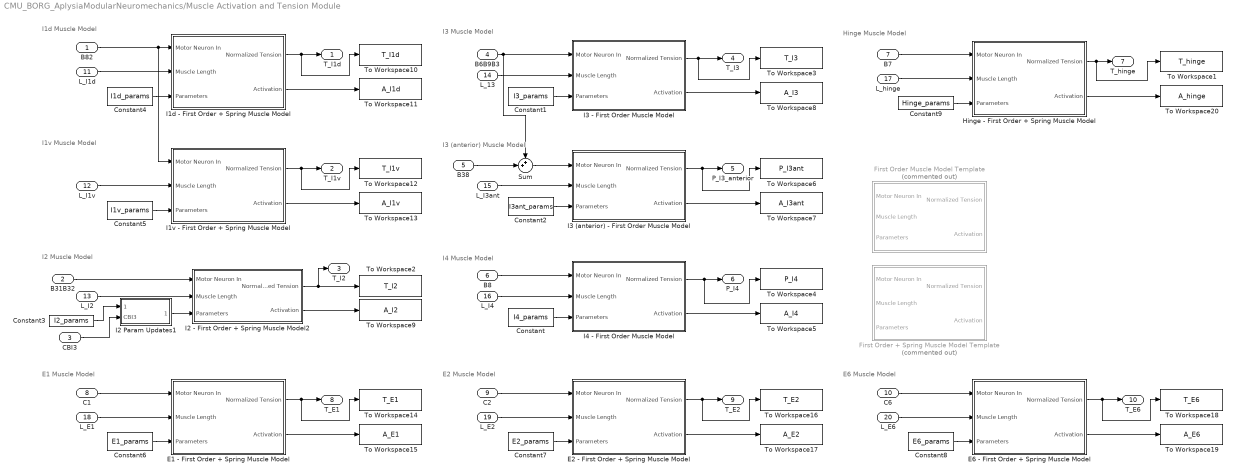
== system CMU_BORG_AplysiaModularNeuromechanics/Muscle Activation and Tension Module ==
  note: I2 Muscle Model
  note: I3 Muscle Model
  note: I3 (anterior) Muscle Model
  note: I4 Muscle Model
  note: Hinge Muscle Model
  note: I1d Muscle Model
  note: I1v Muscle Model
  note: E1 Muscle Model
  note: E2 Muscle Model
  note: E6 Muscle Model
  B82 : Inport
  B31B32 : Inport  Port=2
  CBI3 : Inport  Port=3
  B6B9B3 : Inport  Port=4
  B38 : Inport  Port=5
  B8 : Inport  Port=6
  B7 : Inport  Port=7
  C1 : Inport  Port=8
  C2 : Inport  Port=9
  C6 : Inport  Port=10
  L_I1d : Inport  Port=11
  L_I1v : Inport  Port=12
  L_I2 : Inport  Port=13
  L_13 : Inport  Port=14
  L_I3ant : Inport  Port=15
  L_I4 : Inport  Port=16
  L_hinge : Inport  Port=17
  L_E1 : Inport  Port=18
  L_E2 : Inport  Port=19
  L_E6 : Inport  Port=20
  Constant : Constant  Value=I4_params
  Constant1 : Constant  Value=I3_params
  Constant2 : Constant  Value=I3ant_params
  Constant3 : Constant  Value=I2_params
  Constant4 : Constant  Value=I1d_params
  Constant5 : Constant  Value=I1v_params
  Constant6 : Constant  Value=E1_params
  Constant7 : Constant  Value=E2_params
  Constant8 : Constant  Value=E6_params
  Constant9 : Constant  Value=Hinge_params
  E1 - First Order + Spring Muscle Model : Subsystem
  E2 - First Order + Spring Muscle Model : Subsystem
  E6 - First Order + Spring Muscle Model : Subsystem
  First Order + Spring Muscle Model Template : Subsystem  Commented=on
  First Order Muscle Model Template : Subsystem  Commented=on
  Hinge - First Order + Spring Muscle Model : Subsystem
  I1d - First Order + Spring Muscle Model : Subsystem
  I1v - First Order + Spring Muscle Model : Subsystem
  I2 - First Order + Spring Muscle Model2 : Subsystem
  I2 Param Updates1 : Subsystem
  I3 (anterior) - First Order Muscle Model : Subsystem
  I3 - First Order Muscle Model : Subsystem
  I4 - First Order Muscle Model : Subsystem
  Sum : Sum  Inputs=++|
  To Workspace1 : ToWorkspace  VariableName=T_hinge  SampleTime=-1
  To Workspace10 : ToWorkspace  VariableName=T_I1d  SampleTime=-1
  To Workspace11 : ToWorkspace  VariableName=A_I1d  SampleTime=-1
  To Workspace12 : ToWorkspace  VariableName=T_I1v  SampleTime=-1
  To Workspace13 : ToWorkspace  VariableName=A_I1v  SampleTime=-1
  To Workspace14 : ToWorkspace  VariableName=T_E1  SampleTime=-1
  To Workspace15 : ToWorkspace  VariableName=A_E1  SampleTime=-1
  To Workspace16 : ToWorkspace  VariableName=T_E2  SampleTime=-1
  To Workspace17 : ToWorkspace  VariableName=A_E2  SampleTime=-1
  To Workspace18 : ToWorkspace  VariableName=T_E6  SampleTime=-1
  To Workspace19 : ToWorkspace  VariableName=A_E6  SampleTime=-1
  To Workspace2 : ToWorkspace  VariableName=T_I2  SampleTime=-1
  To Workspace20 : ToWorkspace  VariableName=A_hinge  SampleTime=-1
  To Workspace3 : ToWorkspace  VariableName=T_I3  SampleTime=-1
  To Workspace4 : ToWorkspace  VariableName=P_I4  SampleTime=-1
  To Workspace5 : ToWorkspace  VariableName=A_I4  SampleTime=-1
  To Workspace6 : ToWorkspace  VariableName=P_I3ant  SampleTime=-1
  To Workspace7 : ToWorkspace  VariableName=A_I3ant  SampleTime=-1
  To Workspace8 : ToWorkspace  VariableName=A_I3  SampleTime=-1
  To Workspace9 : ToWorkspace  VariableName=A_I2  SampleTime=-1
  T_I1d : Outport
  T_I1v : Outport  Port=2
  T_I2 : Outport  Port=3
  T_I3 : Outport  Port=4
  P_I3_anterior : Outport  Port=5
  P_I4 : Outport  Port=6
  T_hinge : Outport  Port=7
  T_E1 : Outport  Port=8
  T_E2 : Outport  Port=9
  T_E6 : Outport  Port=10
  wires:
  L_hinge/1 -> Hinge - First Order + Spring Muscle Model/2(Muscle Length)
  L_I4/1 -> I4 - First Order Muscle Model/2(Muscle Length)
  B8/1 -> I4 - First Order Muscle Model/1(Motor Neuron In)
  Constant/1 -> I4 - First Order Muscle Model/3(Parameters)
  B6B9B3/1 -> I3 - First Order Muscle Model/1(Motor Neuron In), Sum/1
  L_13/1 -> I3 - First Order Muscle Model/2(Muscle Length)
  Constant1/1 -> I3 - First Order Muscle Model/3(Parameters)
  B38/1 -> Sum/2
  Sum/1 -> I3 (anterior) - First Order Muscle Model/1(Motor Neuron In)
  L_I3ant/1 -> I3 (anterior) - First Order Muscle Model/2(Muscle Length)
  Constant2/1 -> I3 (anterior) - First Order Muscle Model/3(Parameters)
  I4 - First Order Muscle Model/1(Normalized Tension) -> To Workspace4/1, P_I4/1
  I3 (anterior) - First Order Muscle Model/1(Normalized Tension) -> To Workspace6/1, P_I3_anterior/1
  I3 - First Order Muscle Model/1(Normalized Tension) -> To Workspace3/1, T_I3/1
  I4 - First Order Muscle Model/2(Activation) -> To Workspace5/1
  I3 (anterior) - First Order Muscle Model/2(Activation) -> To Workspace7/1
  I3 - First Order Muscle Model/2(Activation) -> To Workspace8/1
  L_I1d/1 -> I1d - First Order + Spring Muscle Model/2(Muscle Length)
  I1d - First Order + Spring Muscle Model/1(Normalized Tension) -> To Workspace10/1, T_I1d/1
  Constant4/1 -> I1d - First Order + Spring Muscle Model/3(Parameters)
  I1d - First Order + Spring Muscle Model/2(Activation) -> To Workspace11/1
  Constant5/1 -> I1v - First Order + Spring Muscle Model/3(Parameters)
  I1v - First Order + Spring Muscle Model/2(Activation) -> To Workspace13/1
  B82/1 -> I1v - First Order + Spring Muscle Model/1(Motor Neuron In), I1d - First Order + Spring Muscle Model/1(Motor Neuron In)
  I1v - First Order + Spring Muscle Model/1(Normalized Tension) -> To Workspace12/1, T_I1v/1
  L_I1v/1 -> I1v - First Order + Spring Muscle Model/2(Muscle Length)
  E1 - First Order + Spring Muscle Model/2(Activation) -> To Workspace15/1
  Constant6/1 -> E1 - First Order + Spring Muscle Model/3(Parameters)
  C1/1 -> E1 - First Order + Spring Muscle Model/1(Motor Neuron In)
  E1 - First Order + Spring Muscle Model/1(Normalized Tension) -> To Workspace14/1, T_E1/1
  L_E1/1 -> E1 - First Order + Spring Muscle Model/2(Muscle Length)
  E2 - First Order + Spring Muscle Model/2(Activation) -> To Workspace17/1
  Constant7/1 -> E2 - First Order + Spring Muscle Model/3(Parameters)
  C2/1 -> E2 - First Order + Spring Muscle Model/1(Motor Neuron In)
  E2 - First Order + Spring Muscle Model/1(Normalized Tension) -> To Workspace16/1, T_E2/1
  L_E2/1 -> E2 - First Order + Spring Muscle Model/2(Muscle Length)
  C6/1 -> E6 - First Order + Spring Muscle Model/1(Motor Neuron In)
  E6 - First Order + Spring Muscle Model/1(Normalized Tension) -> To Workspace18/1, T_E6/1
  Constant8/1 -> E6 - First Order + Spring Muscle Model/3(Parameters)
  L_E6/1 -> E6 - First Order + Spring Muscle Model/2(Muscle Length)
  E6 - First Order + Spring Muscle Model/2(Activation) -> To Workspace19/1
  B7/1 -> Hinge - First Order + Spring Muscle Model/1(Motor Neuron In)
  Constant9/1 -> Hinge - First Order + Spring Muscle Model/3(Parameters)
  Hinge - First Order + Spring Muscle Model/1(Normalized Tension) -> To Workspace1/1, T_hinge/1
  Hinge - First Order + Spring Muscle Model/2(Activation) -> To Workspace20/1
  Constant3/1 -> I2 Param Updates1/1(In params)
  CBI3/1 -> I2 Param Updates1/2(CBI3)
  B31B32/1 -> I2 - First Order + Spring Muscle Model2/1(Motor Neuron In)
  L_I2/1 -> I2 - First Order + Spring Muscle Model2/2(Muscle Length)
  I2 - First Order + Spring Muscle Model2/1(Normalized Tension) -> T_I2/1, To Workspace2/1
  I2 - First Order + Spring Muscle Model2/2(Activation) -> To Workspace9/1
  I2 Param Updates1/1(Out params) -> I2 - First Order + Spring Muscle Model2/3(Parameters)

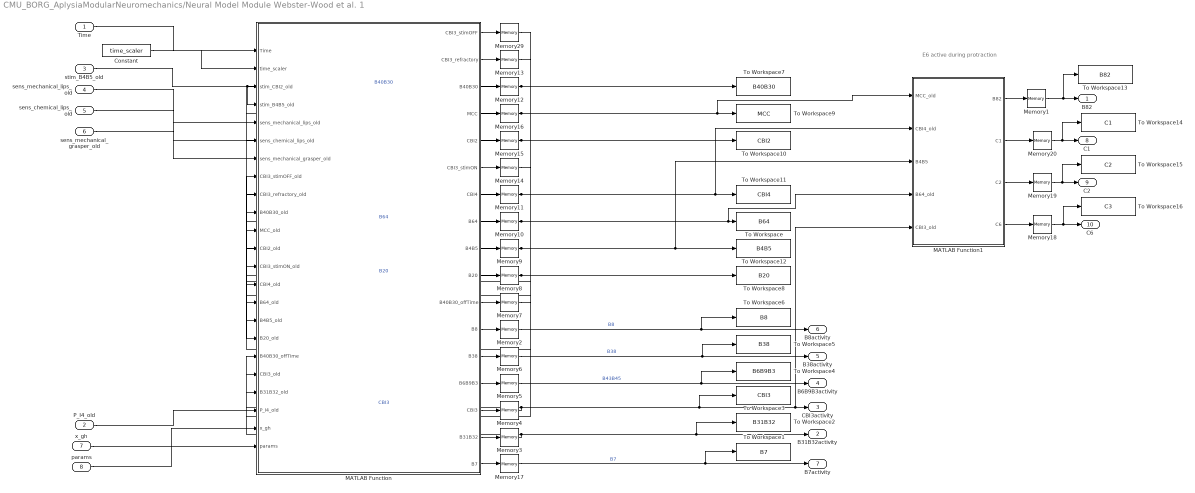
== system CMU_BORG_AplysiaModularNeuromechanics/Neural Model Module Webster-Wood et al. 1 ==
  note: E6 active during protraction
  Time : Inport
  P_I4_old : Inport  Port=2
  stim_B4B5_old : Inport  Port=3
  sens_mechanical_lips_old : Inport  Port=4
  sens_chemical_lips_old : Inport  Port=5
  sens_mechanical_grasper_old : Inport  Port=6
  x_gh : Inport  Port=7
  params : Inport  Port=8
  Constant : Constant  Value=time_scaler
  MATLAB Function : MATLAB Function  TreatAsAtomicUnit=on
  MATLAB Function1 : MATLAB Function  TreatAsAtomicUnit=on
  Memory1 : Memory  InitialCondition=B43B45_0
  Memory10 : Memory  InitialCondition=B64_0
  Memory11 : Memory  InitialCondition=CBI4_0
  Memory12 : Memory  InitialCondition=B40B30_0
  Memory13 : Memory  InitialCondition=CBI3_refractory_0
  Memory14 : Memory  InitialCondition=CBI3_stimON_0
  Memory15 : Memory  InitialCondition=CBI2_0
  Memory16 : Memory  InitialCondition=MCC_0
  Memory17 : Memory  InitialCondition=B7_0
  Memory18 : Memory  InitialCondition=C6_0
  Memory19 : Memory  InitialCondition=C2_0
  Memory2 : Memory  InitialCondition=B8_0
  Memory20 : Memory  InitialCondition=C1_0
  Memory29 : Memory  InitialCondition=CBI3_stimOFF_0
  Memory3 : Memory  InitialCondition=B31B32_0
  Memory4 : Memory  InitialCondition=CBI3_0
  Memory5 : Memory  InitialCondition=B6B9B3_0
  Memory6 : Memory  InitialCondition=B38_0
  Memory7 : Memory  InitialCondition=B40B30_offTime_0
  Memory8 : Memory  InitialCondition=B20_0
  Memory9 : Memory  InitialCondition=B4B5_0
  To Workspace : ToWorkspace  VariableName=B64  SampleTime=-1
  To Workspace1 : ToWorkspace  VariableName=B7  SampleTime=-1
  To Workspace10 : ToWorkspace  VariableName=CBI2  SampleTime=-1
  To Workspace11 : ToWorkspace  VariableName=CBI4  SampleTime=-1
  To Workspace12 : ToWorkspace  VariableName=B4B5  SampleTime=-1
  To Workspace13 : ToWorkspace  VariableName=B82  SampleTime=-1
  To Workspace14 : ToWorkspace  VariableName=C1  SampleTime=-1
  To Workspace15 : ToWorkspace  VariableName=C2  SampleTime=-1
  To Workspace16 : ToWorkspace  VariableName=C3  SampleTime=-1
  To Workspace2 : ToWorkspace  VariableName=B31B32  SampleTime=-1
  To Workspace3 : ToWorkspace  VariableName=CBI3  SampleTime=-1
  To Workspace4 : ToWorkspace  VariableName=B6B9B3  SampleTime=-1
  To Workspace5 : ToWorkspace  VariableName=B38  SampleTime=-1
  To Workspace6 : ToWorkspace  VariableName=B8  SampleTime=-1
  To Workspace7 : ToWorkspace  VariableName=B40B30  SampleTime=-1
  To Workspace8 : ToWorkspace  VariableName=B20  SampleTime=-1
  To Workspace9 : ToWorkspace  VariableName=MCC  SampleTime=-1
  B82 : Outport
  B31B32activity : Outport  Port=2
  CBI3activity : Outport  Port=3
  B6B9B3activity : Outport  Port=4
  B38activity : Outport  Port=5
  B8activity : Outport  Port=6
  B7activity : Outport  Port=7
  C1 : Outport  Port=8
  C2 : Outport  Port=9
  C6 : Outport  Port=10
  wires:
  P_I4_old/1 -> MATLAB Function/21(P_I4_old)
  sens_mechanical_lips_old/1 -> MATLAB Function/5(sens_mechanical_lips_old)
  Time/1 -> MATLAB Function/1(Time)
  sens_mechanical_grasper_old/1 -> MATLAB Function/7(sens_mechanical_grasper_old)
  MATLAB Function/8(B64) -> Memory10/1
  Memory11/1 -> MATLAB Function1/2(CBI4_old), To Workspace11/1, MATLAB Function/14(CBI4_old)
  Memory6/1 -> To Workspace5/1, B38activity/1  "B38"
  Memory2/1 -> To Workspace6/1, B8activity/1  "B8"
  MATLAB Function/12(B8) -> Memory2/1
  sens_chemical_lips_old/1 -> MATLAB Function/6(sens_chemical_lips_old)
  Memory10/1 -> MATLAB Function1/4(B64_old), To Workspace/1, MATLAB Function/15(B64_old)  "B64"
  Memory9/1 -> MATLAB Function1/3(B4B5), To Workspace12/1, MATLAB Function/16(B4B5_old)
  MATLAB Function/3(B40B30) -> Memory12/1
  Memory14/1 -> MATLAB Function/13(CBI3_stimON_old)
  Memory12/1 -> To Workspace7/1, MATLAB Function/10(B40B30_old)  "B40B30"
  MATLAB Function/2(CBI3_refractory) -> Memory13/1
  stim_B4B5_old/1 -> MATLAB Function/3(stim_CBI2_old), MATLAB Function/4(stim_B4B5_old)
  Memory17/1 -> To Workspace1/1, B7activity/1  "B7"
  Memory13/1 -> MATLAB Function/9(CBI3_refractory_old)
  Memory8/1 -> To Workspace8/1, MATLAB Function/17(B20_old)  "B20"
  Memory4/1 -> MATLAB Function/19(CBI3_old), MATLAB Function1/5(CBI3_old), CBI3activity/1, To Workspace3/1  "CBI3"
  Memory15/1 -> To Workspace10/1, MATLAB Function/12(CBI2_old)
  MATLAB Function/9(B4B5) -> Memory9/1
  MATLAB Function/16(B31B32) -> Memory3/1
  MATLAB Function/11(B40B30_offTime) -> Memory7/1
  MATLAB Function/1(CBI3_stimOFF) -> Memory29/1
  MATLAB Function/6(CBI3_stimON) -> Memory14/1
  MATLAB Function/7(CBI4) -> Memory11/1
  MATLAB Function/14(B6B9B3) -> Memory5/1
  MATLAB Function/13(B38) -> Memory6/1
  MATLAB Function/10(B20) -> Memory8/1
  Memory7/1 -> MATLAB Function/18("B40B30_offTime ")
  MATLAB Function/15(CBI3) -> Memory4/1
  Memory16/1 -> MATLAB Function1/1(MCC_old), To Workspace9/1, MATLAB Function/11(MCC_old)
  x_gh/1 -> MATLAB Function/22(x_gh)
  MATLAB Function/5(CBI2) -> Memory15/1
  Memory29/1 -> MATLAB Function/8(CBI3_stimOFF_old)
  MATLAB Function/17(B7) -> Memory17/1
  MATLAB Function/4(MCC) -> Memory16/1
  MATLAB Function1/1(B82) -> Memory1/1
  MATLAB Function1/4(C6) -> Memory18/1
  Memory18/1 -> To Workspace16/1, C6/1
  MATLAB Function1/3(C2) -> Memory19/1
  MATLAB Function1/2(C1) -> Memory20/1
  Memory20/1 -> To Workspace14/1, C1/1
  Memory19/1 -> To Workspace15/1, C2/1
  Memory5/1 -> B6B9B3activity/1, To Workspace4/1  "B43B45"
  Memory1/1 -> To Workspace13/1, B82/1
  Constant/1 -> MATLAB Function/2(time_scaler)
  Memory3/1 -> MATLAB Function/20(B31B32_old), B31B32activity/1, To Workspace2/1
  params/1 -> MATLAB Function/23(params)

== system CMU_BORG_AplysiaModularNeuromechanics/Subsystem ==
  Time : Inport
  Constant : Constant  Value=t_switch_mech_lips
  Constant1 : Constant  Value=sens_mechanical_lips
  GreaterThan : RelationalOperator  Operator=>  OutDataTypeStr=boolean  RndMeth=Simplest  InputSameDT=off
  NOT : Logic  Operator=NOT  IconShape=distinctive  AllPortsSameDT=off  OutDataTypeStr=boolean
  Switch : Switch  Criteria=u2 > Threshold  SaturateOnIntegerOverflow=off  InputSameDT=off
  sens_mechanical_lips_old : Outport
  wires:
  Time/1 -> GreaterThan/1
  Constant/1 -> GreaterThan/2
  GreaterThan/1 -> Switch/2
  Constant1/1 -> NOT/1, Switch/3
  NOT/1 -> Switch/1
  Switch/1 -> sens_mechanical_lips_old/1

== system CMU_BORG_AplysiaModularNeuromechanics/Subsystem1 ==
  Time : Inport
  Constant : Constant  Value=t_switch_chem_lips
  Constant1 : Constant  Value=sens_chemical_lips
  GreaterThan : RelationalOperator  Operator=>  OutDataTypeStr=boolean  RndMeth=Simplest  InputSameDT=off
  NOT : Logic  Operator=NOT  IconShape=distinctive  AllPortsSameDT=off  OutDataTypeStr=boolean
  Switch : Switch  Criteria=u2 > Threshold  SaturateOnIntegerOverflow=off  InputSameDT=off
  sens_chemical_lips_old : Outport
  wires:
  Time/1 -> GreaterThan/1
  Constant/1 -> GreaterThan/2
  GreaterThan/1 -> Switch/2
  Constant1/1 -> NOT/1, Switch/3
  NOT/1 -> Switch/1
  Switch/1 -> sens_chemical_lips_old/1

== system CMU_BORG_AplysiaModularNeuromechanics/Subsystem2 ==
  Time : Inport
  Constant : Constant  Value=t_switch_mech_grasp
  Constant1 : Constant  Value=sens_mechanical_grasper
  GreaterThan : RelationalOperator  Operator=>  OutDataTypeStr=boolean  RndMeth=Simplest  InputSameDT=off
  NOT : Logic  Operator=NOT  IconShape=distinctive  AllPortsSameDT=off  OutDataTypeStr=boolean
  Switch : Switch  Criteria=u2 > Threshold  SaturateOnIntegerOverflow=off  InputSameDT=off
  sens_mechanical_grasper_old : Outport
  wires:
  Time/1 -> GreaterThan/1
  Constant/1 -> GreaterThan/2
  GreaterThan/1 -> Switch/2
  Constant1/1 -> NOT/1, Switch/3
  NOT/1 -> Switch/1
  Switch/1 -> sens_mechanical_grasper_old/1

== system CMU_BORG_AplysiaModularNeuromechanics/Subsystem3 ==
  note: if the chemical sensation is gone, the unfix the seaweed so length can be calculated
  Time : Inport
  sens_chemical_lips_old : Inport  Port=2
  AND : Logic  IconShape=distinctive  AllPortsSameDT=off  OutDataTypeStr=boolean
  Constant : Constant  Value=t_switch_fixation
  Constant1 : Constant  Value=fixation_type
  GreaterThan : RelationalOperator  Operator=>  OutDataTypeStr=boolean  RndMeth=Simplest  InputSameDT=off
  NOT : Logic  Operator=NOT  IconShape=distinctive  AllPortsSameDT=off  OutDataTypeStr=boolean
  Scope : Scope  NumInputPorts=2
  Switch : Switch  Criteria=u2 > Threshold  SaturateOnIntegerOverflow=off  InputSameDT=off
  fixation : Outport
  wires:
  Time/1 -> GreaterThan/1
  Constant/1 -> GreaterThan/2
  GreaterThan/1 -> Scope/2, Switch/2
  Constant1/1 -> NOT/1, Switch/3
  NOT/1 -> Switch/1
  AND/1 -> Scope/1, fixation/1
  Switch/1 -> AND/1
  sens_chemical_lips_old/1 -> AND/2
